simulink model "sim1_3"  (R2017b)
settings: Solver=ode5  StartTime=0.0  StopTime=50  FixedStep=0.001  RelTol=1e-3
settings Model: Creator=kiran  LastModifiedBy=kiran

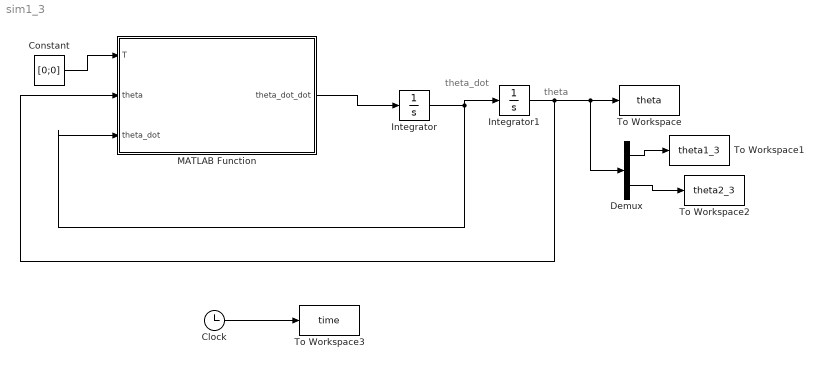
== system sim1_3 ==
  note: theta
  note: theta_dot
  Clock : Clock
  Constant : Constant  Value=[0;0]
  Demux : Demux  Outputs=2
  Integrator : Integrator  InitialCondition=[0;0]
  Integrator1 : Integrator  InitialCondition=[pi/3.00001;0]
  MATLAB Function : MATLAB Function  TreatAsAtomicUnit=on
  To Workspace : ToWorkspace  VariableName=theta  SampleTime=-1
  To Workspace1 : ToWorkspace  VariableName=theta1_3  SampleTime=-1
  To Workspace2 : ToWorkspace  VariableName=theta2_3  SampleTime=-1
  To Workspace3 : ToWorkspace  VariableName=time  SampleTime=-1
  wires:
  MATLAB Function/1(theta_dot_dot) -> Integrator/1
  Integrator/1 -> MATLAB Function/3(theta_dot), Integrator1/1
  Integrator1/1 -> MATLAB Function/2(theta), Demux/1, To Workspace/1
  Constant/1 -> MATLAB Function/1(T)
  Demux/1 -> To Workspace1/1
  Demux/2 -> To Workspace2/1
  Clock/1 -> To Workspace3/1

== matlab function sim1_3/MATLAB Function ==
  data: T input; theta_dot_dot output; theta input; theta_dot input
function theta_dot_dot = fcn(T,theta,theta_dot)
l1 =0.5;    %m
l2 = 0.3;   %m
r1 = 0.25;  %m
r2 = 0.15;  %m
m1 = 0.5;   %kg
m2 = 0.3;   %kg
I1 = 0.0104;%kg-m^2
I2 = 0.0022;%kg-m^2
c1 = 0;     %N.m.s/rad
c2 = 0;     %N.m.s/rad
g = 9.81;   %m/s^2

alpha = I1+I2+m1*r1^2+m2*(l1^2+r2^2);
beta = m2*l1*r2;
gamma = I2+m2*r2^2;

theta1 = theta(1);
theta2 = theta(2);
theta1_dot = theta_dot(1);
theta2_dot = theta_dot(2);

M =[alpha+2*beta.*cos(theta2) gamma+beta.*cos(theta2); gamma+beta.*cos(theta2) gamma];
C = [c1-beta.*theta2_dot.*sin(theta2) -beta.*(theta1_dot+theta2_dot).*sin(theta2); beta*theta1_dot.*sin(theta2) c2];
N = [(m1*r1+m2*l1)*g.*cos(theta1)+m2*r2*g.*cos(theta1+theta2); m2*r2*g.*cos(theta1+theta2)];

theta_dot_dot = inv(M)*(T-C*theta_dot-N);
end
